simulink model "modelo_lti_aumentado_sim"  (R2023b)
settings: Solver=VariableStepAuto  StartTime=0.0  StopTime=1  MaxStep=1e-4  RelTol=1e-3
values from neighbouring files (symbols this model uses):
  b_eq = b_eq_max    (= 2.40277777778e-05)    [analisis_estabilidad.m]    (also in parametros.m = 2.19444444444e-05; parametros_sim.m = 2.19444444444e-05)
  C_ts = 0.818    [analisis_estabilidad.m]    (also in parametros.m; parametros_sim.m)
  J_eq = J_eq_max    (= 4.58263888889e-05)    [analisis_estabilidad.m]    (also in parametros.m = 1.97847222222e-05; parametros_sim.m = 1.97847222222e-05)
  L_d = 6.6    [analisis_estabilidad.m]    (also in parametros.m = 0.0066; parametros_sim.m; polosyceros.m = L_d^3)
  L_ls = 0.8    [analisis_estabilidad.m]    (also in parametros.m = 0.0008; parametros_sim.m)
  L_q = 5.8    [analisis_estabilidad.m]    (also in parametros.m = 0.0058; parametros_sim.m; polosyceros.m = L_q^3)
  lambda_m = 0.016    [analisis_estabilidad.m]    (also in parametros.m; parametros_sim.m)
  P_p = 3    [analisis_estabilidad.m]    (also in parametros.m; parametros_sim.m)
  r = 120    [analisis_estabilidad.m]    (also in parametros.m; parametros_sim.m)
  R_s = R_s_max    (= 1.39791)    [analisis_estabilidad.m]    (also in frec_nat_y_amort.m = R_s_ref * (1 + alpha_Cu * (T - T_s_ref)); parametros.m = 1.02)
  R_ts_amb = 146.7    [analisis_estabilidad.m]    (also in parametros.m; parametros_sim.m)
  T_s_ref = 20    [analisis_estabilidad.m]    (also in parametros.m; parametros_sim.m)
libraries: SignalEditorBlockLib x4
settings Model: Creator=martinarobyculasso  LastModifiedBy=Marti
settings OptimizationCC: ReuseModelBlockBuffer=off

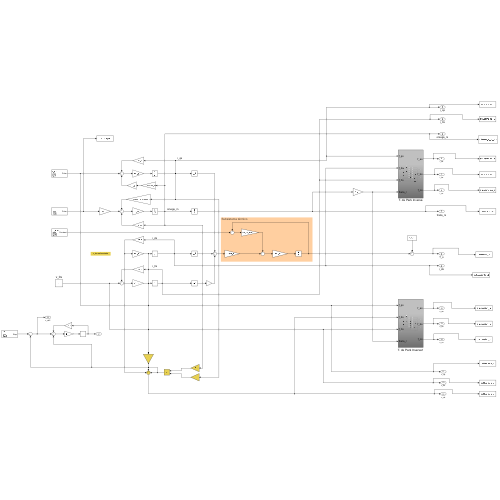
[thumbnail: Simulink's stored preview of the top-level diagram]
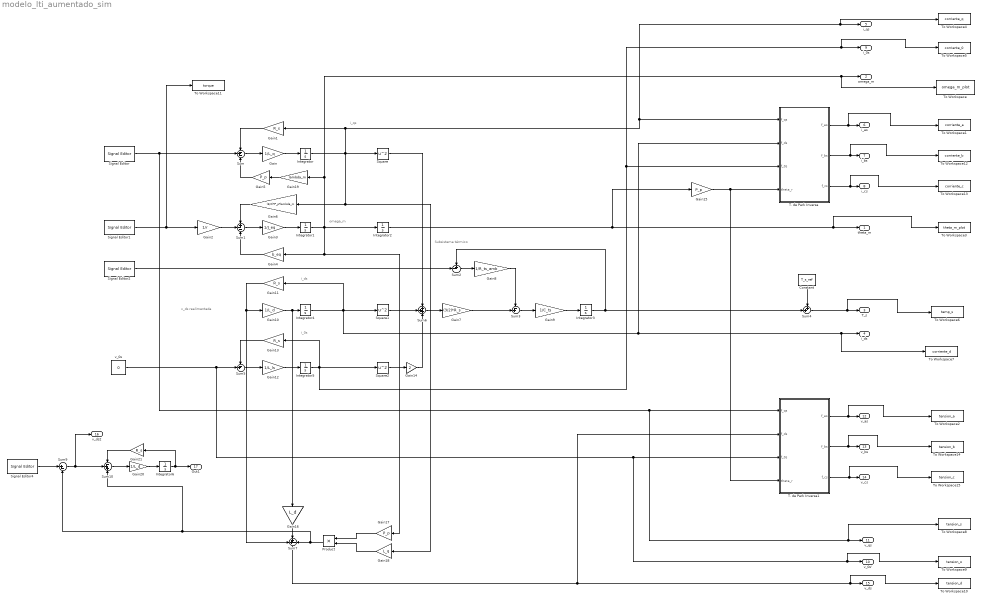
== system modelo_lti_aumentado_sim ==
  note: v_ds realimentada
  note: Subsistema térmico
  note: i_qs
  note: i_0s
  note: i_ds
  note: omega_m
  Constant : Constant  Value=T_s_ref
  Gain : Gain  Gain=1/L_q
  Gain{1,11,13,21} (4 alike) : Gain  Gain=R_s
  Gain10 : Gain  Gain=1/L_d
  Gain12 : Gain  Gain=1/L_ls
  Gain14 : Gain  Gain=2
  Gain15 : Gain  Gain=P_p
  Gain16 : Gain  Gain=L_d
  Gain17 : Gain  Gain=P_p
  Gain18 : Gain  Gain=L_q
  Gain19 : Gain  Gain=lambda_m
  Gain2 : Gain  Gain=1/r
  Gain20 : Gain  Gain=1/L_d
  Gain3 : Gain  Gain=1/J_eq
  Gain4 : Gain  Gain=b_eq
  Gain5 : Gain  Gain=P_p
  Gain6 : Gain  Gain=(3/2)*P_p*lambda_m
  Gain7 : Gain  Gain=(3/2)*R_s
  Gain8 : Gain  Gain=1/R_ts_amb
  Gain9 : Gain  Gain=1/C_ts
  Integrator{,1..6} (7 alike) : Integrator
  Product : Product
  Signal Editor : SignalEditorBlockLib/Signal Editor  FileName=vqs.mat  ActiveScenario=v_qs  ActiveSignal=Pulse  IsBus=off  OutputBusObjectStr=Bus: BusObject  SampleTime=0  Interpolate=off  ZeroCross=off  OutputAfterFinalValue=Setting to zero  Unit=inherit  PreserveSignalName=on  ApplySigPropsToAllScenarios=on  ApplySigPropsToAllSignals=off
  Signal Editor1 : SignalEditorBlockLib/Signal Editor  FileName=tl.mat  ActiveScenario=T_l  ActiveSignal=Pulse  IsBus=off  OutputBusObjectStr=Bus: BusObject  SampleTime=0  Interpolate=off  ZeroCross=off  OutputAfterFinalValue=Setting to zero  Unit=inherit  PreserveSignalName=on  ApplySigPropsToAllScenarios=on  ApplySigPropsToAllSignals=off
  Signal Editor2 : SignalEditorBlockLib/Signal Editor  FileName=tamb.mat  ActiveScenario=T_amb  ActiveSignal=Constant  IsBus=off  OutputBusObjectStr=Bus: BusObject  SampleTime=0  Interpolate=off  ZeroCross=off  OutputAfterFinalValue=Setting to zero  Unit=inherit  PreserveSignalName=on  ApplySigPropsToAllScenarios=on  ApplySigPropsToAllSignals=off
  Signal Editor4 : SignalEditorBlockLib/Signal Editor  FileName=vds2.mat  ActiveScenario=vds  ActiveSignal=Step  IsBus=off  OutputBusObjectStr=Bus: BusObject  SampleTime=0  Interpolate=off  ZeroCross=off  OutputAfterFinalValue=Setting to zero  Unit=inherit  PreserveSignalName=on  ApplySigPropsToAllScenarios=on  ApplySigPropsToAllSignals=off
  Square : Math  Operator=square
  Square1 : Math  Operator=square
  Square2 : Math  Operator=square
  Sum : Sum  Inputs=-+-
  Sum1 : Sum  Inputs=+--
  Sum10 : Sum  Inputs=-++
  Sum2 : Sum  Inputs=+-|
  Sum3 : Sum  Inputs=-+|
  Sum4 : Sum  Inputs=++|
  Sum5 : Sum  Inputs=-+|
  Sum6 : Sum  Inputs=+++
  Sum7 : Sum  Inputs=++-
  Sum9 : Sum  Inputs=|+-
  T. de Park Inversa : Subsystem
  T. de Park Inversa1 : Subsystem
  To Workspace : ToWorkspace  VariableName=omega_m_plot  SaveFormat=Timeseries  SampleTime=-1
  To Workspace1 : ToWorkspace  VariableName=corriente_a  SaveFormat=Timeseries  SampleTime=-1
  To Workspace10 : ToWorkspace  VariableName=tension_d  SaveFormat=Timeseries  SampleTime=-1
  To Workspace11 : ToWorkspace  VariableName=torque  SaveFormat=Timeseries  SampleTime=-1
  To Workspace12 : ToWorkspace  VariableName=corriente_b  SaveFormat=Timeseries  SampleTime=-1
  To Workspace13 : ToWorkspace  VariableName=corriente_c  SaveFormat=Timeseries  SampleTime=-1
  To Workspace14 : ToWorkspace  VariableName=tension_b  SaveFormat=Timeseries  SampleTime=-1
  To Workspace15 : ToWorkspace  VariableName=tension_c  SaveFormat=Timeseries  SampleTime=-1
  To Workspace2 : ToWorkspace  VariableName=tension_a  SaveFormat=Timeseries  SampleTime=-1
  To Workspace3 : ToWorkspace  VariableName=theta_m_plot  SaveFormat=Timeseries  SampleTime=-1
  To Workspace4 : ToWorkspace  VariableName=corriente_q  SaveFormat=Timeseries  SampleTime=-1
  To Workspace5 : ToWorkspace  VariableName=corriente_0  SaveFormat=Timeseries  SampleTime=-1
  To Workspace6 : ToWorkspace  VariableName=temp_s  SaveFormat=Timeseries  SampleTime=-1
  To Workspace7 : ToWorkspace  VariableName=corriente_d  SaveFormat=Timeseries  SampleTime=-1
  To Workspace8 : ToWorkspace  VariableName=tension_s  SaveFormat=Timeseries  SampleTime=-1
  To Workspace9 : ToWorkspace  VariableName=tension_o  SaveFormat=Timeseries  SampleTime=-1
  v_0s : Constant  Value=0
  theta_m : Outport
  omega_m : Outport  Port=2
  T_s : Outport  Port=3
  i_ds : Outport  Port=4
  i_qs : Outport  Port=5
  i_as : Outport  Port=6
  i_bs : Outport  Port=7
  i_cs : Outport  Port=8
  i_0s : Outport  Port=9
  v_0s' : Outport  Port=10
  v_qs : Outport  Port=11
  v_as : Outport  Port=12
  v_bs : Outport  Port=13
  v_cs : Outport  Port=14
  v_ds : Outport  Port=15
  v_ds2 : Outport  Port=16
  Out1 : Outport  Port=17
  wires:
  Sum/1 -> Gain/1
  Gain/1 -> Integrator/1
  Gain1/1 -> Sum/1
  Integrator/1 -> Square/1, Gain6/1, Gain18/1, Gain1/1, T. de Park Inversa/1(f_qs), To Workspace4/1, i_qs/1
  Gain2/1 -> Sum1/2
  Sum1/1 -> Gain3/1
  Gain3/1 -> Integrator1/1
  Integrator1/1 -> Gain17/1, Gain4/1, Gain19/1, To Workspace/1, omega_m/1, Integrator2/1
  Integrator2/1 -> Gain15/1, To Workspace3/1, theta_m/1
  Gain4/1 -> Sum1/3
  Gain5/1 -> Sum/3
  Gain6/1 -> Sum1/1
  Integrator4/1 -> Gain11/1, T. de Park Inversa/2(f_ds), To Workspace7/1, i_ds/1, Square1/1
  Integrator5/1 -> T. de Park Inversa/3(f_0s), To Workspace5/1, i_0s/1, Square2/1, Gain13/1
  Gain12/1 -> Integrator5/1
  v_0s/1 -> To Workspace9/1, v_0s'/1, T. de Park Inversa1/3(f_0s), Sum5/2
  Sum5/1 -> Gain12/1
  Gain13/1 -> Sum5/1
  Sum6/1 -> Gain7/1
  Square1/1 -> Sum6/2
  Square2/1 -> Gain14/1
  Gain14/1 -> Sum6/3
  Square/1 -> Sum6/1
  Sum2/1 -> Gain8/1
  Gain7/1 -> Sum3/2
  Gain8/1 -> Sum3/1
  Sum3/1 -> Gain9/1
  Gain9/1 -> Integrator3/1
  Integrator3/1 -> Sum4/2, Sum2/1
  Signal Editor1/1 -> To Workspace11/1, Gain2/1
  Signal Editor2/1 -> Sum2/2
  Signal Editor/1 -> Sum/2, To Workspace8/1, v_qs/1, T. de Park Inversa1/1(f_qs)
  Gain15/1 -> T. de Park Inversa1/4(theta_r), T. de Park Inversa/4(theta_r)
  T. de Park Inversa/1(f_as) -> To Workspace1/1, i_as/1
  T. de Park Inversa/2(f_bs) -> To Workspace12/1, i_bs/1
  T. de Park Inversa/3(f_cs) -> To Workspace13/1, i_cs/1
  Sum4/1 -> To Workspace6/1, T_s/1
  Constant/1 -> Sum4/1
  T. de Park Inversa1/1(f_as) -> To Workspace2/1, v_as/1
  T. de Park Inversa1/2(f_bs) -> To Workspace14/1, v_bs/1
  T. de Park Inversa1/3(f_cs) -> To Workspace15/1, v_cs/1
  Gain10/1 -> Integrator4/1, Gain16/1
  Gain11/1 -> Sum7/1, Gain10/1
  Gain16/1 -> Sum7/2
  Product/1 -> Sum10/3, Sum9/2, Sum7/3
  Gain18/1 -> Product/2
  Gain17/1 -> Product/1
  Sum7/1 -> T. de Park Inversa1/2(f_ds), To Workspace10/1, v_ds/1
  Gain19/1 -> Gain5/1
  Sum9/1 -> v_ds2/1, Sum10/2
  Signal Editor4/1 -> Sum9/1
  Sum10/1 -> Gain20/1
  Gain20/1 -> Integrator6/1
  Integrator6/1 -> Gain21/1, Out1/1
  Gain21/1 -> Sum10/1

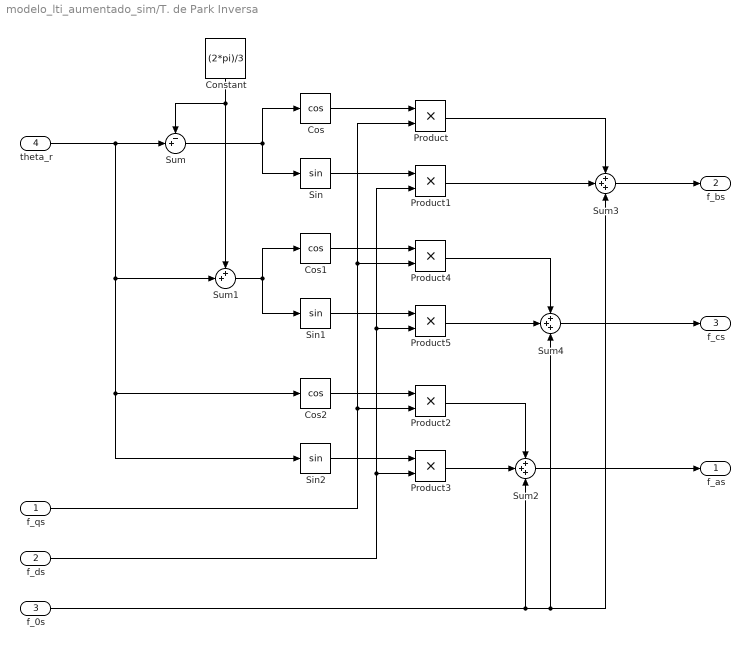
== system modelo_lti_aumentado_sim/T. de Park Inversa ==
  f_qs : Inport
  f_ds : Inport  Port=2
  f_0s : Inport  Port=3
  theta_r : Inport  Port=4
  Constant : Constant  Value=(2*pi)/3
  Cos : Trigonometry  Operator=cos
  Cos1 : Trigonometry  Operator=cos
  Cos2 : Trigonometry  Operator=cos
  Product{,1..5} (6 alike) : Product
  Sin : Trigonometry
  Sin1 : Trigonometry
  Sin2 : Trigonometry
  Sum : Sum  Inputs=-+|
  Sum1 : Sum  Inputs=++|
  Sum2 : Sum  Inputs=+++
  Sum3 : Sum  Inputs=+++
  Sum4 : Sum  Inputs=+++
  f_as : Outport
  f_bs : Outport  Port=2
  f_cs : Outport  Port=3
  wires:
  Product4/1 -> Sum4/1
  Sum2/1 -> f_as/1
  f_qs/1 -> Product4/2, Product/2, Product2/2
  Sum/1 -> Sin/1, Cos/1
  theta_r/1 -> Sum1/2, Cos2/1, Sin2/1, Sum/2
  Product1/1 -> Sum3/2
  Product3/1 -> Sum2/2
  Product5/1 -> Sum4/2
  Sin1/1 -> Product5/1
  Product/1 -> Sum3/1
  Cos/1 -> Product/1
  Sin2/1 -> Product3/1
  Cos1/1 -> Product4/1
  Sin/1 -> Product1/1
  f_0s/1 -> Sum3/3, Sum4/3, Sum2/3
  Sum3/1 -> f_bs/1
  Sum1/1 -> Sin1/1, Cos1/1
  Cos2/1 -> Product2/1
  Product2/1 -> Sum2/1
  Sum4/1 -> f_cs/1
  f_ds/1 -> Product3/2, Product5/2, Product1/2
  Constant/1 -> Sum/1, Sum1/1

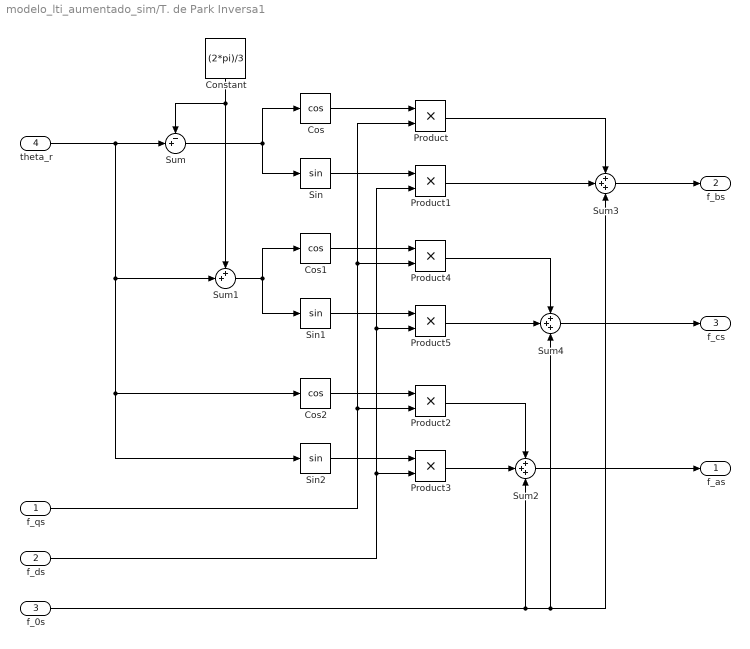
== system modelo_lti_aumentado_sim/T. de Park Inversa1 ==
  f_qs : Inport
  f_ds : Inport  Port=2
  f_0s : Inport  Port=3
  theta_r : Inport  Port=4
  Constant : Constant  Value=(2*pi)/3
  Cos : Trigonometry  Operator=cos
  Cos1 : Trigonometry  Operator=cos
  Cos2 : Trigonometry  Operator=cos
  Product{,1..5} (6 alike) : Product
  Sin : Trigonometry
  Sin1 : Trigonometry
  Sin2 : Trigonometry
  Sum : Sum  Inputs=-+|
  Sum1 : Sum  Inputs=++|
  Sum2 : Sum  Inputs=+++
  Sum3 : Sum  Inputs=+++
  Sum4 : Sum  Inputs=+++
  f_as : Outport
  f_bs : Outport  Port=2
  f_cs : Outport  Port=3
  wires:
  Product4/1 -> Sum4/1
  Sum2/1 -> f_as/1
  f_qs/1 -> Product4/2, Product/2, Product2/2
  Sum/1 -> Sin/1, Cos/1
  theta_r/1 -> Sum1/2, Cos2/1, Sin2/1, Sum/2
  Product1/1 -> Sum3/2
  Product3/1 -> Sum2/2
  Product5/1 -> Sum4/2
  Sin1/1 -> Product5/1
  Product/1 -> Sum3/1
  Cos/1 -> Product/1
  Sin2/1 -> Product3/1
  Cos1/1 -> Product4/1
  Sin/1 -> Product1/1
  f_0s/1 -> Sum3/3, Sum4/3, Sum2/3
  Sum3/1 -> f_bs/1
  Sum1/1 -> Sin1/1, Cos1/1
  Cos2/1 -> Product2/1
  Product2/1 -> Sum2/1
  Sum4/1 -> f_cs/1
  f_ds/1 -> Product3/2, Product5/2, Product1/2
  Constant/1 -> Sum/1, Sum1/1
